simulink model "Linear_Moving_Setpoint_SS_Int"  (R2022a)
settings: Solver=VariableStepAuto  StartTime=tspan(1)  StopTime=tspan(2)  RelTol=1e-9
undefined symbols (not defined in the file): K1, K2, r_sim
settings Model: Creator=domin  LastModifiedBy=domin
settings SolverCC: AlgebraicLoopSolver=TrustRegion
settings DebuggingCC: AlgebraicLoopMsg=none  UnconnectedInputMsg=warning  UnconnectedOutputMsg=warning  UnconnectedLineMsg=warning  SFMachineParentedDataDiag=warning
settings RTWCC: DLArmComputeVersion=19.05

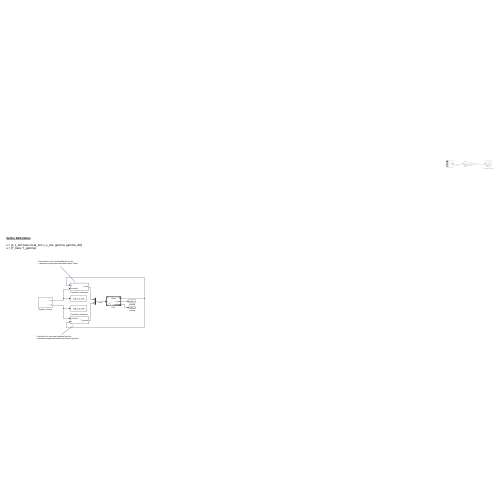
[thumbnail: Simulink's stored preview of the top-level diagram]
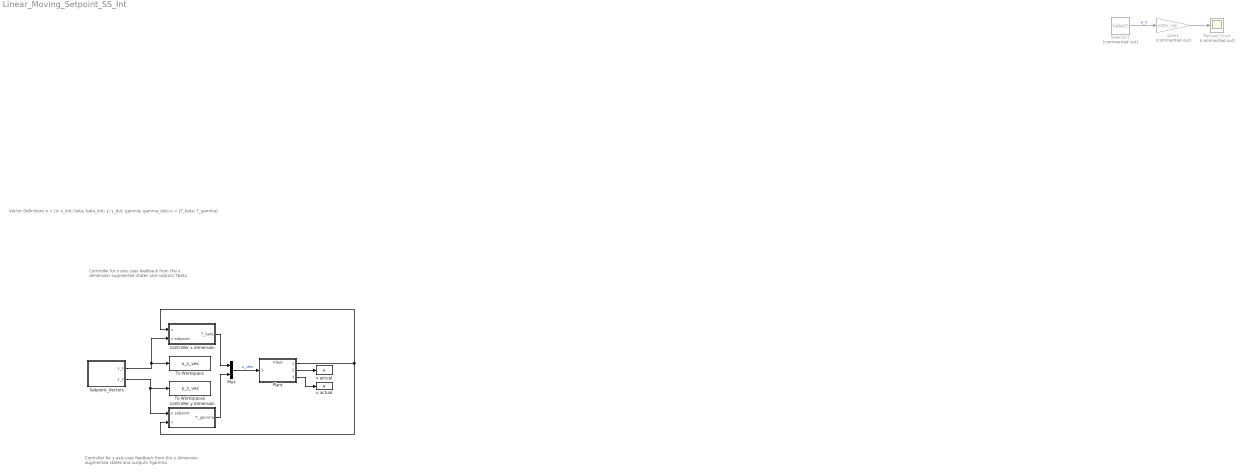
== system Linear_Moving_Setpoint_SS_Int ==
  note: Controller for y axis uses feedback from the
      | y dimension augmented states and outputs Tgamma
  note: Controller for x axis uses feedback from the
      | x dimension augmented states and outputs Tbeta
  note: Vector Definitions
      |
      | x = [x; x_dot; beta; beta_dot; y; y_dot; gamma; gamma_dot]
      | u = [T_beta; T_gamma]
  Controller x dimension : Subsystem
  Controller y dimension : Subsystem
  Gain5 : Gain  Commented=on  Gain=100/r_sim
  Mux : Mux  Inputs=2
  Percent Error : Scope  Commented=on
  Plant : ModelReference  ModelNameDialog=Plant  SimulationMode=Normal  ModelReferenceVersion=1.107
  Selector1 : Selector  Commented=on  InputPortWidth=5  IndexOptions=Index vector (dialog)  Indices=[1]  OutputSizes=1
  Setpoint_Vectors : Subsystem
  To Workspace : ToWorkspace  VariableName=x_s_vec  SampleTime=-1
  To Workspace2 : ToWorkspace  VariableName=y_s_vec  SampleTime=-1
  u actual : ToWorkspace  VariableName=u  SampleTime=-1
  x actual : ToWorkspace  VariableName=x  SampleTime=-1
  wires:
  Gain5/1 -> Percent Error/1
  Selector1/1 -> Gain5/1  "e_x"
  Controller x dimension/1(T_beta) -> Mux/1
  Controller y dimension/1(T_gamma) -> Mux/2
  Plant/1 -> Controller x dimension/1(x), Controller y dimension/2(x)
  Mux/1 -> Plant/1  "u_des"
  Plant/2 -> x actual/1
  Plant/3 -> u actual/1
  Setpoint_Vectors/2(y_s) -> Controller y dimension/1(y setpoint), To Workspace2/1
  Setpoint_Vectors/1(x_s) -> Controller x dimension/2(x setpoint), To Workspace/1

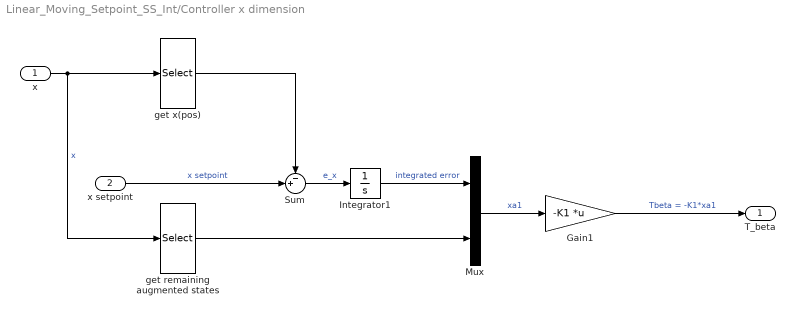
== system Linear_Moving_Setpoint_SS_Int/Controller x dimension ==
  x : Inport
  x setpoint : Inport  Port=2
  Gain1 : Gain  Gain=-K1  Multiplication=Matrix(K*u)
  Integrator1 : Integrator
  Mux : Mux  Inputs=2
  Sum : Sum  Inputs=-+|
  get remaining augmented states : Selector  InputPortWidth=8  IndexOptions=Index vector (dialog)  Indices=[1,2,3,4]  OutputSizes=1
  get x(pos) : Selector  InputPortWidth=8  IndexOptions=Index vector (dialog)  Indices=[1]  OutputSizes=1
  T_beta : Outport
  wires:
  get remaining augmented states/1 -> Mux/2
  Gain1/1 -> T_beta/1  "Tbeta = -K1*xa1"
  get x(pos)/1 -> Sum/1
  Mux/1 -> Gain1/1  "xa1"
  Sum/1 -> Integrator1/1  "e_x"
  Integrator1/1 -> Mux/1  "integrated error"
  x setpoint/1 -> Sum/2  "x setpoint"
  x/1 -> get remaining augmented states/1, get x(pos)/1  "x"

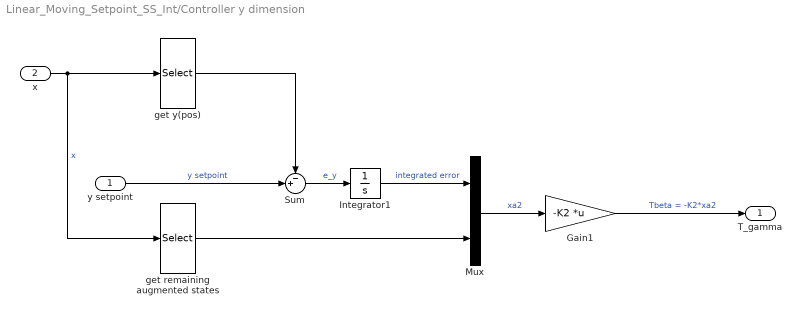
== system Linear_Moving_Setpoint_SS_Int/Controller y dimension ==
  y setpoint : Inport
  x : Inport  Port=2
  Gain1 : Gain  Gain=-K2  Multiplication=Matrix(K*u)
  Integrator1 : Integrator
  Mux : Mux  Inputs=2
  Sum : Sum  Inputs=-+|
  get remaining augmented states : Selector  InputPortWidth=8  IndexOptions=Index vector (dialog)  Indices=[5,6,7,8]  OutputSizes=1
  get y(pos) : Selector  InputPortWidth=8  IndexOptions=Index vector (dialog)  Indices=[2]  OutputSizes=1
  T_gamma : Outport
  wires:
  x/1 -> get y(pos)/1, get remaining augmented states/1  "x"
  y setpoint/1 -> Sum/2  "y setpoint"
  Integrator1/1 -> Mux/1  "integrated error"
  Sum/1 -> Integrator1/1  "e_y"
  Mux/1 -> Gain1/1  "xa2"
  get y(pos)/1 -> Sum/1
  Gain1/1 -> T_gamma/1  "Tbeta = -K2*xa2"
  get remaining augmented states/1 -> Mux/2

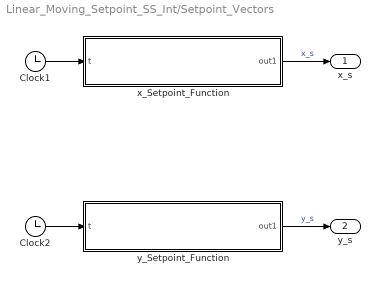
== system Linear_Moving_Setpoint_SS_Int/Setpoint_Vectors ==
  Clock1 : Clock
  Clock2 : Clock
  x_Setpoint_Function : MATLAB Function  TreatAsAtomicUnit=on
  y_Setpoint_Function : MATLAB Function  TreatAsAtomicUnit=on
  x_s : Outport
  y_s : Outport  Port=2
  wires:
  y_Setpoint_Function/1(out1) -> y_s/1  "y_s"
  Clock2/1 -> y_Setpoint_Function/1(t)
  Clock1/1 -> x_Setpoint_Function/1(t)
  x_Setpoint_Function/1(out1) -> x_s/1  "x_s"

== matlab function Linear_Moving_Setpoint_SS_Int/Setpoint_Vectors/y_Setpoint_Function ==
  data: t input; out1 output
function out1 = y_s_vec(t)
%#codegen

%    This function was generated by the Symbolic Math Toolbox version 9.1.
%    18-Apr-2022 12:08:24

t2 = t./2.0;
t3 = -t2;
t4 = exp(t3);
out1 = t4.*(3.0./2.0e+1)-sin((t.*pi)./3.0).*(t4-1.0).*(3.0./1.0e+1);

== matlab function Linear_Moving_Setpoint_SS_Int/Setpoint_Vectors/x_Setpoint_Function ==
  data: t input; out1 output
function out1 = x_s_vec(t)
%#codegen

%    This function was generated by the Symbolic Math Toolbox version 9.1.
%    18-Apr-2022 12:08:22

t2 = t./2.0;
t3 = -t2;
t4 = exp(t3);
out1 = t4.*(3.0./2.0e+1)-sin((t.*pi)./3.0).*(t4-1.0).*(3.0./1.0e+1);
